simulink model "pedestrian"  (R2022a)
settings: Solver=VariableStepAuto  StartTime=0.0  StopTime=10.0  RelTol=1e-3
settings Model: Creator=Taha  LastModifiedBy=Asus
settings SolverCC: AlgebraicLoopSolver=TrustRegion
settings DebuggingCC: UnconnectedInputMsg=warning  UnconnectedOutputMsg=warning  UnconnectedLineMsg=warning  SFMachineParentedDataDiag=warning
settings RTWCC: DLArmComputeVersion=19.05

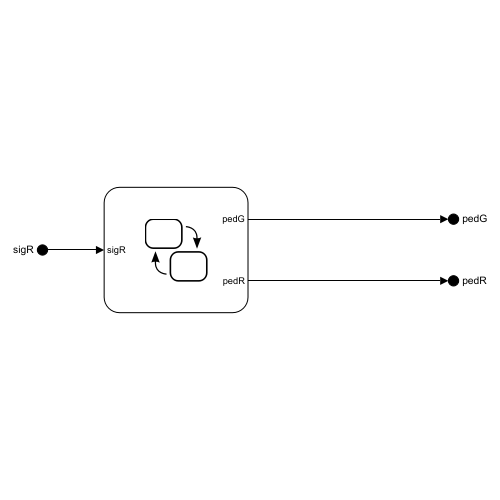
[thumbnail: Simulink's stored preview of the top-level diagram]
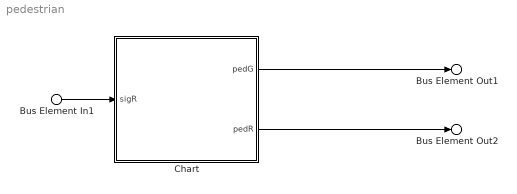
== system pedestrian ==
  Bus Element In1 : Inport  PortName=sigR
  Chart : Stateflow chart  TreatAsAtomicUnit=on
  Bus Element Out1 : Outport  PortName=pedG
  Bus Element Out2 : Outport  Port=2  PortName=pedR
  wires:
  Bus Element In1/1 -> Chart/1(sigR)
  Chart/1(pedG) -> Bus Element Out1/1
  Chart/2(pedR) -> Bus Element Out2/1

== stateflow chart pedestrian/Chart ==
  state green
  state red
  green -> red [order 1] : [pcount>=55]
      | {pedR=1;}
  (default) -> green : {pcount=0;}
  red -> green : [sigR==1]
      | {pedG=1;pcount=0;}
  green -> green [order 2] : {pcount=pcount+1;}
  data: sigR input; pedG output; pedR output; pcount local
